simulink model "quadcopter_dynamics2"  (R2020a)
settings: Solver=ode45  StartTime=0.0  StopTime=30  FixedStep=0.001  MinStep=0.01
PreLoadFcn:
  | 
  | initialization;
undefined symbols (not defined in the file or in its folder): Parameter
libraries: eeGeneralControl x10
settings Model: Creator=salva  LastModifiedBy=salva
settings SolverCC: MaxConsecutiveMinStep=auto
settings DataIOCC: ExternalInput=[t]

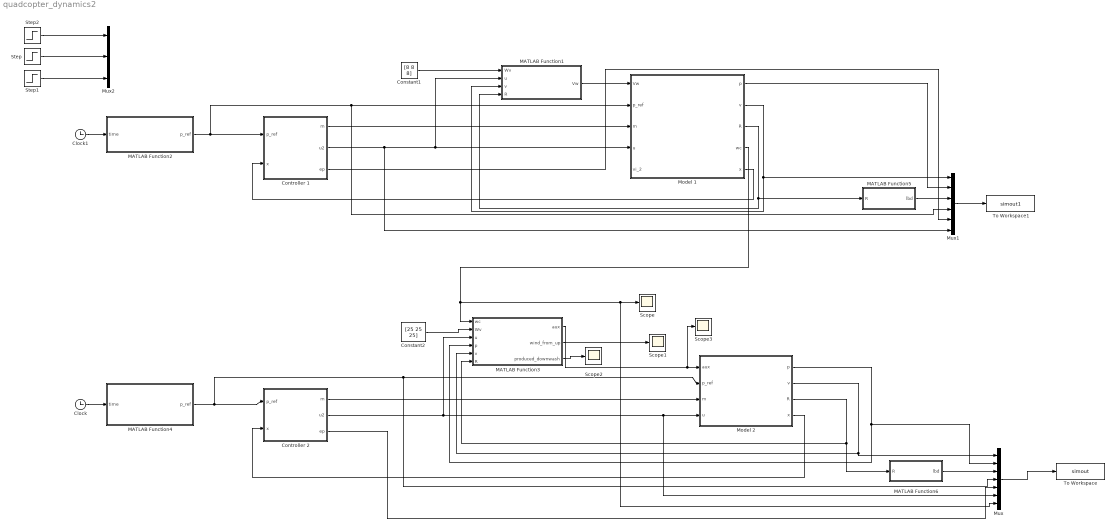
== system quadcopter_dynamics2 ==
  Clock : Clock
      settings: Decimation=50
  Clock1 : Clock
      settings: Decimation=50
  Constant1 : Constant  Value=[8 8 8]
  Constant2 : Constant  Value=[25 25 25]
  Controller 1 : Subsystem
  Controller 2 : Subsystem
  MATLAB Function1 : MATLAB Function  TreatAsAtomicUnit=on
  MATLAB Function2 : MATLAB Function  TreatAsAtomicUnit=on
  MATLAB Function3 : MATLAB Function  TreatAsAtomicUnit=on
  MATLAB Function4 : MATLAB Function  TreatAsAtomicUnit=on
  MATLAB Function5 : MATLAB Function  TreatAsAtomicUnit=on
  MATLAB Function6 : MATLAB Function  TreatAsAtomicUnit=on
  Model 1 : Subsystem
  Model 2 : Subsystem
  Mux : Mux  Inputs=7
  Mux1 : Mux  Inputs=6
  Mux2 : Mux  Inputs=3
  Scope{,1..3} (4 alike) : Scope
  Step : Step  Time=2  After=4  SampleTime=0
  Step1 : Step  Time=2  After=4  SampleTime=0
  Step2 : Step  Time=2  After=4  SampleTime=0
  To Workspace : ToWorkspace  VariableName=simout  SaveFormat=Timeseries  SampleTime=-1
  To Workspace1 : ToWorkspace  VariableName=simout1  SaveFormat=Timeseries  SampleTime=-1
  wires:
  Mux/1 -> To Workspace/1
  Clock/1 -> MATLAB Function4/1(time)
  Model 2/2(v) -> MATLAB Function3/5(v), Mux/1
  Model 2/1(p) -> MATLAB Function3/4(p), Mux/2
  Model 2/3(R) -> MATLAB Function3/6(R), MATLAB Function6/1(R)
  Controller 2/2(u2) -> MATLAB Function3/3(u), Model 2/4(u), Mux/6
  Controller 2/1(m) -> Model 2/3(m)
  Controller 2/3(ep) -> Mux/5
  Controller 1/1(m) -> Model 1/3(m)
  Model 1/1(p) -> Mux1/2
  Controller 1/2(u2) -> MATLAB Function1/2(u), Model 1/4(u), Mux1/6
  Model 1/2(v) -> MATLAB Function1/3(v), Mux1/1
  MATLAB Function1/1(Vw) -> Model 1/1(Vw)
  Model 1/3(R) -> MATLAB Function1/4(R), MATLAB Function5/1(R)
  Controller 1/3(ep) -> Mux1/5
  Clock1/1 -> MATLAB Function2/1(time)
  Mux1/1 -> To Workspace1/1
  MATLAB Function3/1(aux) -> Scope3/1, Model 2/1(aux)
  Constant1/1 -> MATLAB Function1/1(Wv)
  Constant2/1 -> MATLAB Function3/2(Wv)
  MATLAB Function3/2(wind_from_up) -> Scope1/1
  MATLAB Function3/3(produced_downwash) -> Scope2/1
  Model 1/5(x) -> Controller 1/2(x)
  MATLAB Function5/1(lbd) -> Mux1/3
  Model 2/4(x) -> Controller 2/2(x)
  MATLAB Function6/1(lbd) -> Mux/3
  Model 1/4(wc) -> Mux/7, Scope/1, MATLAB Function3/1(wc)
  Step/1 -> Mux2/2
  Step2/1 -> Mux2/1
  Step1/1 -> Mux2/3
  MATLAB Function2/1(p_ref) -> Controller 1/1(p_ref), Model 1/2(p_ref), Mux1/4
  MATLAB Function4/1(p_ref) -> Mux/4, Model 2/2(p_ref), Controller 2/1(p_ref)

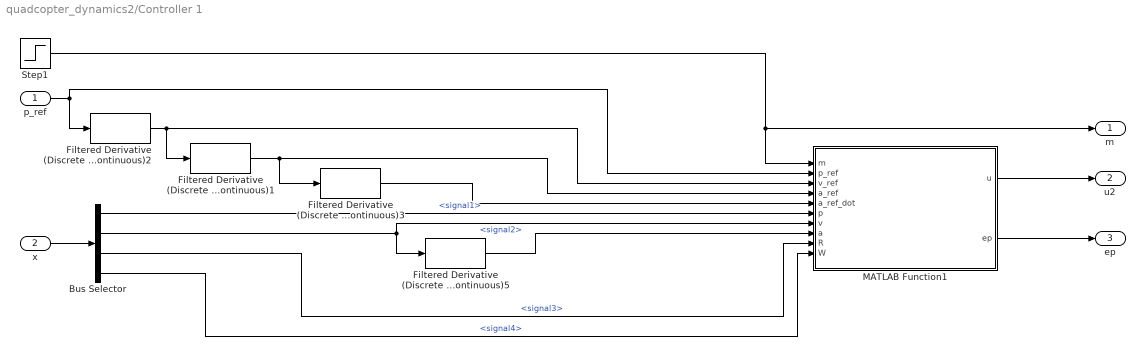
== system quadcopter_dynamics2/Controller 1 ==
  p_ref : Inport
  x : Inport  Port=2
  Bus Selector : BusSelector  OutputSignals=signal1,signal2,signal3,signal4
  Filtered Derivative (Discrete or Continuous){1..3,5} (4 alike) : eeGeneralControl/Filtered Derivative (Discrete or Continuous)  K=1  T=0.001  B=inf  A=-inf  minRatio=10  init_option=Inherited from block input  x0=0  Ts=-1
      settings: SourceProductBaseCode=PS
  MATLAB Function1 : MATLAB Function  TreatAsAtomicUnit=on
  Step1 : Step  Time=15  Before=4  After=6  SampleTime=0
  m : Outport
  u2 : Outport  Port=2
  ep : Outport  Port=3
  wires:
  Filtered Derivative (Discrete or Continuous)3/1 -> MATLAB Function1/5(a_ref_dot)
  Filtered Derivative (Discrete or Continuous)5/1 -> MATLAB Function1/8(a)
  Filtered Derivative (Discrete or Continuous)2/1 -> Filtered Derivative (Discrete or Continuous)1/1, MATLAB Function1/3(v_ref)
  Filtered Derivative (Discrete or Continuous)1/1 -> Filtered Derivative (Discrete or Continuous)3/1, MATLAB Function1/4(a_ref)
  Step1/1 -> MATLAB Function1/1(m), m/1
  Bus Selector/2 -> Filtered Derivative (Discrete or Continuous)5/1, MATLAB Function1/7(v)  "<signal2>"
  Bus Selector/1 -> MATLAB Function1/6(p)  "<signal1>"
  MATLAB Function1/2(ep) -> ep/1
  p_ref/1 -> Filtered Derivative (Discrete or Continuous)2/1, MATLAB Function1/2(p_ref)
  MATLAB Function1/1(u) -> u2/1
  Bus Selector/3 -> MATLAB Function1/9(R)  "<signal3>"
  Bus Selector/4 -> MATLAB Function1/10(W)  "<signal4>"
  x/1 -> Bus Selector/1

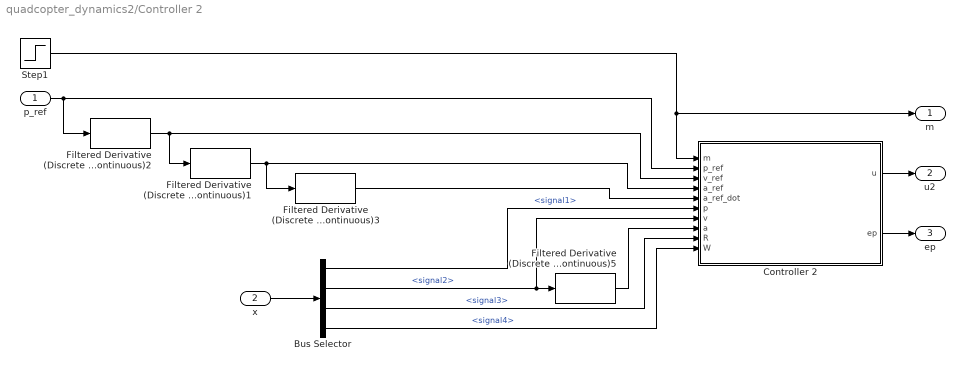
== system quadcopter_dynamics2/Controller 2 ==
  p_ref : Inport
  x : Inport  Port=2
  Bus Selector : BusSelector  OutputSignals=signal1,signal2,signal3,signal4
  Controller 2 : MATLAB Function  TreatAsAtomicUnit=on
  Filtered Derivative (Discrete or Continuous){1..3,5} (4 alike) : eeGeneralControl/Filtered Derivative (Discrete or Continuous)  K=1  T=0.001  B=inf  A=-inf  minRatio=10  init_option=Inherited from block input  x0=0  Ts=-1
      settings: SourceProductBaseCode=PS
  Step1 : Step  Time=15  Before=4  After=6  SampleTime=0
  m : Outport
  u2 : Outport  Port=2
  ep : Outport  Port=3
  wires:
  Filtered Derivative (Discrete or Continuous)3/1 -> Controller 2/5(a_ref_dot)
  Filtered Derivative (Discrete or Continuous)5/1 -> Controller 2/8(a)
  Filtered Derivative (Discrete or Continuous)2/1 -> Filtered Derivative (Discrete or Continuous)1/1, Controller 2/3(v_ref)
  Filtered Derivative (Discrete or Continuous)1/1 -> Filtered Derivative (Discrete or Continuous)3/1, Controller 2/4(a_ref)
  Step1/1 -> Controller 2/1(m), m/1
  Bus Selector/2 -> Controller 2/7(v), Filtered Derivative (Discrete or Continuous)5/1  "<signal2>"
  Bus Selector/1 -> Controller 2/6(p)  "<signal1>"
  Controller 2/2(ep) -> ep/1
  p_ref/1 -> Filtered Derivative (Discrete or Continuous)2/1, Controller 2/2(p_ref)
  Controller 2/1(u) -> u2/1
  Bus Selector/3 -> Controller 2/9(R)  "<signal3>"
  Bus Selector/4 -> Controller 2/10(W)  "<signal4>"
  x/1 -> Bus Selector/1

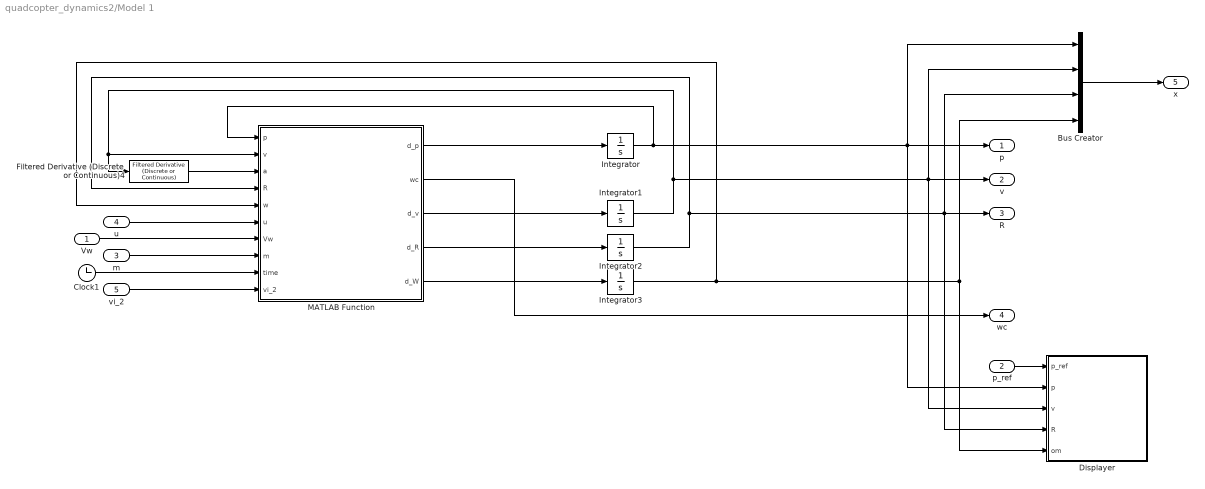
== system quadcopter_dynamics2/Model 1 ==
  Vw : Inport
  p_ref : Inport  Port=2
  m : Inport  Port=3
  u : Inport  Port=4
  vi_2 : Inport  Port=5
  Bus Creator : BusCreator  Inputs=4
  Clock1 : Clock
      settings: Decimation=50
  Displayer : Subsystem
  Filtered Derivative (Discrete or Continuous)4 : eeGeneralControl/Filtered Derivative (Discrete or Continuous)  K=1  T=0.01  B=inf  A=-inf  minRatio=10  init_option=Inherited from block input  x0=0  Ts=-1
      settings: SourceProductBaseCode=PS
  Integrator : Integrator  InitialCondition=Parameter.p_initial_2
  Integrator1 : Integrator  InitialCondition=Parameter.v_initial
  Integrator2 : Integrator  InitialCondition=Parameter.R_initial
  Integrator3 : Integrator  InitialCondition=Parameter.omega_initial
  MATLAB Function : MATLAB Function  TreatAsAtomicUnit=on
  p : Outport
  v : Outport  Port=2
  R : Outport  Port=3
  wc : Outport  Port=4
  x : Outport  Port=5
  wires:
  Clock1/1 -> MATLAB Function/9(time)
  Filtered Derivative (Discrete or Continuous)4/1 -> MATLAB Function/3(a)
  Integrator2/1 -> Bus Creator/3, Displayer/4(R), R/1, MATLAB Function/4(R)
  MATLAB Function/3(d_v) -> Integrator1/1
  MATLAB Function/5(d_W) -> Integrator3/1
  MATLAB Function/1(d_p) -> Integrator/1
  Integrator3/1 -> Bus Creator/4, Displayer/5(om), MATLAB Function/5(w)
  MATLAB Function/4(d_R) -> Integrator2/1
  Integrator1/1 -> Bus Creator/2, Displayer/3(v), v/1, Filtered Derivative (Discrete or Continuous)4/1, MATLAB Function/2(v)
  u/1 -> MATLAB Function/6(u)
  p_ref/1 -> Displayer/1(p_ref)
  Integrator/1 -> MATLAB Function/1(p), Bus Creator/1, p/1, Displayer/2(p)
  m/1 -> MATLAB Function/8(m)
  Vw/1 -> MATLAB Function/7(Vw)
  MATLAB Function/2(wc) -> wc/1
  vi_2/1 -> MATLAB Function/10(vi_2)
  Bus Creator/1 -> x/1

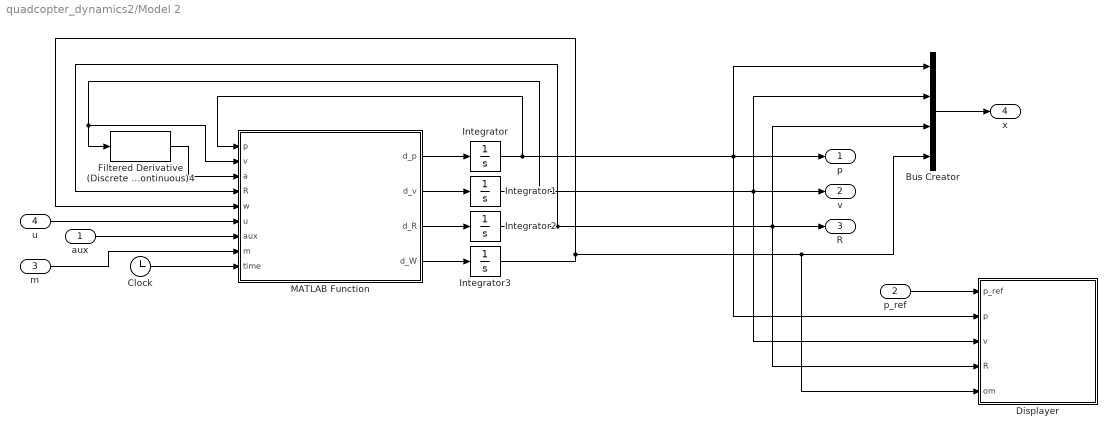
== system quadcopter_dynamics2/Model 2 ==
  aux : Inport
  p_ref : Inport  Port=2
  m : Inport  Port=3
  u : Inport  Port=4
  Bus Creator : BusCreator  Inputs=4
  Clock : Clock
      settings: Decimation=50
  Displayer : Subsystem
  Filtered Derivative (Discrete or Continuous)4 : eeGeneralControl/Filtered Derivative (Discrete or Continuous)  K=1  T=0.01  B=inf  A=-inf  minRatio=10  init_option=Inherited from block input  x0=0  Ts=-1
      settings: SourceProductBaseCode=PS
  Integrator : Integrator  InitialCondition=Parameter.p_initial_1
  Integrator1 : Integrator  InitialCondition=Parameter.v_initial
  Integrator2 : Integrator  InitialCondition=Parameter.R_initial
  Integrator3 : Integrator  InitialCondition=Parameter.omega_initial
  MATLAB Function : MATLAB Function  TreatAsAtomicUnit=on
  p : Outport
  v : Outport  Port=2
  R : Outport  Port=3
  x : Outport  Port=4
  wires:
  Clock/1 -> MATLAB Function/9(time)
  Filtered Derivative (Discrete or Continuous)4/1 -> MATLAB Function/3(a)
  MATLAB Function/2(d_v) -> Integrator1/1
  MATLAB Function/4(d_W) -> Integrator3/1
  MATLAB Function/1(d_p) -> Integrator/1
  Integrator2/1 -> MATLAB Function/4(R), Bus Creator/3, Displayer/4("R "), R/1
  MATLAB Function/3(d_R) -> Integrator2/1
  u/1 -> MATLAB Function/6(u)
  p_ref/1 -> Displayer/1(p_ref)
  Integrator/1 -> Bus Creator/1, Displayer/2(p), p/1, MATLAB Function/1(p)
  Integrator1/1 -> Bus Creator/2, Displayer/3(v), v/1, Filtered Derivative (Discrete or Continuous)4/1, MATLAB Function/2(v)
  m/1 -> MATLAB Function/8(m)
  aux/1 -> MATLAB Function/7(aux)
  Integrator3/1 -> Bus Creator/4, Displayer/5(om), MATLAB Function/5(w)
  Bus Creator/1 -> x/1

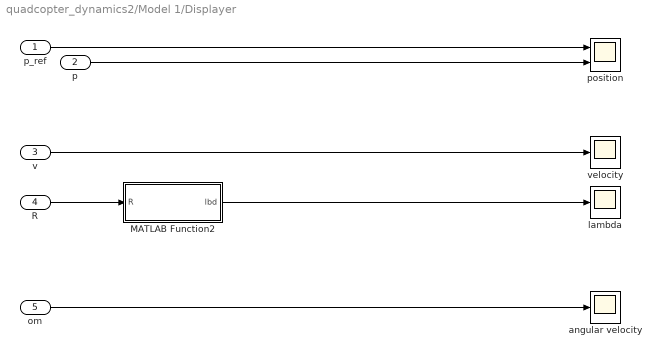
== system quadcopter_dynamics2/Model 1/Displayer ==
  p_ref : Inport
  p : Inport  Port=2
  v : Inport  Port=3
  R : Inport  Port=4
  om : Inport  Port=5
  MATLAB Function2 : MATLAB Function  TreatAsAtomicUnit=on
  angular velocity : Scope
  lambda : Scope
  position : Scope  NumInputPorts=2
  velocity : Scope
  wires:
  p/1 -> position/2
  v/1 -> velocity/1
  p_ref/1 -> position/1
  om/1 -> angular velocity/1
  R/1 -> MATLAB Function2/1(R)
  MATLAB Function2/1(lbd) -> lambda/1

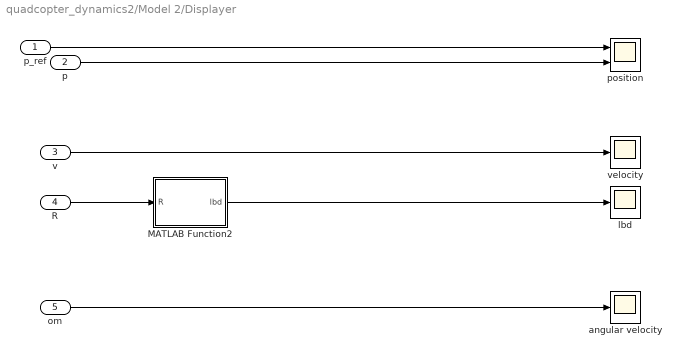
== system quadcopter_dynamics2/Model 2/Displayer ==
  p_ref : Inport
  p : Inport  Port=2
  v : Inport  Port=3
  "R " : Inport  Port=4
  om : Inport  Port=5
  MATLAB Function2 : MATLAB Function  TreatAsAtomicUnit=on
  angular velocity : Scope
  lbd : Scope
  position : Scope  NumInputPorts=2
  velocity : Scope
  wires:
  p/1 -> position/2
  v/1 -> velocity/1
  p_ref/1 -> position/1
  om/1 -> angular velocity/1
  "R "/1 -> MATLAB Function2/1(R)
  MATLAB Function2/1(lbd) -> lbd/1

== matlab function quadcopter_dynamics2/MATLAB Function2 ==
  data: p_ref output; time input; Parameter parameter



function p_ref = reference_values(time, Parameter)


P = Parameter;
 z_ref = 0;
 y_ref = 0;
 x_ref = 0;
switch P.trajectory_2
    case  1
        z_ref = 3;
        y_ref = 2*sin(sqrt(2)*time)*cos(sqrt(2)*time);
        x_ref = 2*cos(sqrt(2)*time);
        
 
    case 4
      
        z_ref =exp((0.5*(time-15)^2)/5^2)+ 2.60 + P.height;
        y_ref = 3;
        x_ref = time;
        

         
        
end

 
p_ref = [x_ref;y_ref;z_ref];

== matlab function quadcopter_dynamics2/Model 1/MATLAB Function ==
  data: p input; v input; a input; R input; w input; u input; d_p output; wc output; d_v output; Parameter parameter; Vw input; m input; d_R output; d_W output; time input; vi_2 input
function [d_p,wc,d_v,d_R,d_W]= quad_model(p,v,a,R,w,u,Parameter,Vw,m,time,vi_2)
%QUADROTOR_MODEL Summary of this function goes here

[d_p,wc,d_v,d_R,d_W]= quadcopter_model1(p,v,a,R,w,u,Parameter,Vw,m,time,vi_2);

== matlab function quadcopter_dynamics2/MATLAB Function5 ==
  data: R input; lbd output
function lbd = R_to_Euler(R)
%   lbd = R2euler(R)  ,  with  R in SO(3)
%   lbd in R^3 is the vector of the Z-Y-X euler angles that define R
%
    lbd = zeros(3,1);
    lbd(2,1) = atan2(-R(3,1),sqrt(R(1,1)^2 + R(2,1)^2));
    if abs(cos(lbd(2,1))) < eps %if it is a singular configuration
        lbd(3,1) = 0; %Yaw
        lbd(1,1) = sign(lbd(2,1))*atan2(R(1,2),R(2,2)); %Roll
    else
        lbd(3,1) = atan2(R(2,1)/cos(lbd(2)),R(1,1)/cos(lbd(2))); %Yaw
        lbd(1,1) = atan2(R(3,2)/cos(lbd(2)),R(3,3)/cos(lbd(2))); %Roll
    end
    
end

== matlab function quadcopter_dynamics2/Controller 1/MATLAB Function1 ==
  data: m input; p_ref input; v_ref input; a_ref input; a_ref_dot input; Parameter parameter; p input; u output; v input; a input; R input; W input; ep output
 function [u,ep] = slx_quad_controller(m,p_ref,v_ref,a_ref,a_ref_dot,Parameter,p,v,a,R,W)
%QUADROTOR_CONTROLLER Summary of this function goes here

[u,ep] = quadcopter_controller1(m,p_ref,v_ref,a_ref,a_ref_dot,Parameter,p,v,a,R,W);

== matlab function quadcopter_dynamics2/Model 1/Displayer/MATLAB Function2 ==
  data: R input; lbd output
function lbd = R_to_Euler(R)
%   lbd = R2euler(R)  ,  with  R in SO(3)
%   lbd in R^3 is the vector of the Z-Y-X euler angles that define R
%
    lbd = zeros(3,1);
    lbd(2,1) = atan2(-R(3,1),sqrt(R(1,1)^2 + R(2,1)^2));
    if abs(cos(lbd(2,1))) < eps %if it is a singular configuration
        lbd(3,1) = 0; %Yaw
        lbd(1,1) = sign(lbd(2,1))*atan2(R(1,2),R(2,2)); %Roll
    else
        lbd(3,1) = atan2(R(2,1)/cos(lbd(2)),R(1,1)/cos(lbd(2))); %Yaw
        lbd(1,1) = atan2(R(3,2)/cos(lbd(2)),R(3,3)/cos(lbd(2))); %Roll
    end
    
end

== matlab function quadcopter_dynamics2/MATLAB Function6 ==
  data: R input; lbd output
function lbd = R_to_Euler(R)
%   lbd = R2euler(R)  ,  with  R in SO(3)
%   lbd in R^3 is the vector of the Z-Y-X euler angles that define R
%
    lbd = zeros(3,1);
    lbd(2,1) = atan2(-R(3,1),sqrt(R(1,1)^2 + R(2,1)^2));
    if abs(cos(lbd(2,1))) < eps %if it is a singular configuration
        lbd(3,1) = 0; %Yaw
        lbd(1,1) = sign(lbd(2,1))*atan2(R(1,2),R(2,2)); %Roll
    else
        lbd(3,1) = atan2(R(2,1)/cos(lbd(2)),R(1,1)/cos(lbd(2))); %Yaw
        lbd(1,1) = atan2(R(3,2)/cos(lbd(2)),R(3,3)/cos(lbd(2))); %Roll
    end
    
end

== matlab function quadcopter_dynamics2/Controller 2/Controller 2 ==
  data: m input; p_ref input; v_ref input; a_ref input; a_ref_dot input; Parameter parameter; p input; u output; v input; a input; R input; W input; ep output
 function [u,ep]   = quad_control2(m,p_ref,v_ref,a_ref, a_ref_dot,Parameter,p,v,a,R,W)
%QUADROTOR_CONTROLLER Summary of this function goes here

[u,ep] = quadcopter_controller2(m, p,p_ref,v_ref,a_ref, a_ref_dot, Parameter,v,a,R,W);

== matlab function quadcopter_dynamics2/Model 2/MATLAB Function ==
  data: p input; v input; a input; R input; w input; u input; d_p output; d_v output; Parameter parameter; aux input; m input; d_R output; d_W output; time input
function [d_p,d_v,d_R,d_W]= quad_model2(p,v,a,R,w,u,Parameter,aux,m,time)
%QUADROTOR_MODEL Summary of this function goes here

[d_p,d_v,d_R,d_W]= quadcopter_model2(p,v,a,R,w,u,Parameter,aux,m,time);

== matlab function quadcopter_dynamics2/Model 2/Displayer/MATLAB Function2 ==
  data: R input; lbd output
function lbd = R_to_Euler(R)
%   lbd = R2euler(R)  ,  with  R in SO(3)
%   lbd in R^3 is the vector of the Z-Y-X euler angles that define R
%
    lbd = zeros(3,1);
    lbd(2,1) = atan2(-R(3,1),sqrt(R(1,1)^2 + R(2,1)^2));
    if abs(cos(lbd(2,1))) < eps %if it is a singular configuration
        lbd(3,1) = 0; %Yaw
        lbd(1,1) = sign(lbd(2,1))*atan2(R(1,2),R(2,2)); %Roll
    else
        lbd(3,1) = atan2(R(2,1)/cos(lbd(2)),R(1,1)/cos(lbd(2))); %Yaw
        lbd(1,1) = atan2(R(3,2)/cos(lbd(2)),R(3,3)/cos(lbd(2))); %Roll
    end
    
end

== matlab function quadcopter_dynamics2/MATLAB Function3 ==
  data: wc input; Wv input; u input; p input; aux output; v input; R input; Parameter parameter; wind_from_up output; produced_downwash output
function [aux, wind_from_up, produced_downwash]  = wind_model(wc,Wv,u,p,v,R,Parameter)

[aux, wind_from_up, produced_downwash]  = wind_model2(Wv,u,v,wc, R,p,Parameter);

== matlab function quadcopter_dynamics2/MATLAB Function4 ==
  data: p_ref output; time input; Parameter parameter



function p_ref   = reference_values(time, Parameter)


P = Parameter;
  
 z_ref = 0;
 y_ref = 0;
 x_ref = 0;

switch P.trajectory
    case  1
        z_ref = 3;
        y_ref = 2*sin(sqrt(2)*time)*cos(sqrt(2)*time);
        x_ref = 2*cos(sqrt(2)*time);
        
    case 2
        z_ref = 3;
        y_ref = 2*sin(sqrt(2)*time);
        x_ref = 2*cos(sqrt(2)*time);
    case 3
        z_ref = time;
        y_ref = 2*sin(time);
        x_ref = 2*cos(time);
        
    case 4
        z_ref = 3;
        y_ref = 3;
        x_ref =  time;
        

         
        
end

 
p_ref = [x_ref;y_ref;z_ref];

== matlab function quadcopter_dynamics2/MATLAB Function1 ==
  data: Wv input; u input; Vw output; v input; R input; Parameter parameter
function Vw  = slx_wind_model(Wv,u,v,R,Parameter)

Vw  = wind_model1(Wv,u,v,R,Parameter)
